simulink model "dirdyna_OffRoadRobot"  (Simulink 8.1)
settings: Solver=ode45  StartTime=0.0  StopTime=10.0  MaxStep=1e-2  RelTol=1e-3  AbsTol=1e-6
undefined symbols (not defined in the file or in its folder): Function_dirdynared, MBStoAnimFile_StopFcnCallback, Modules, Robotran, S
settings Model: Creator=habra  LastModifiedBy=habra
settings SolverCC: InitialStep=1e-3
settings DataIOCC: SignalLoggingSaveFormat=Dataset
settings OptimizationCC: ExpressionDepthLimit=128
settings DebuggingCC: FcnCallInpInsideContextMsg=EnableAllAsError
settings GRTTargetCC: CombineOutputUpdateFcns=on  GRTInterface=off

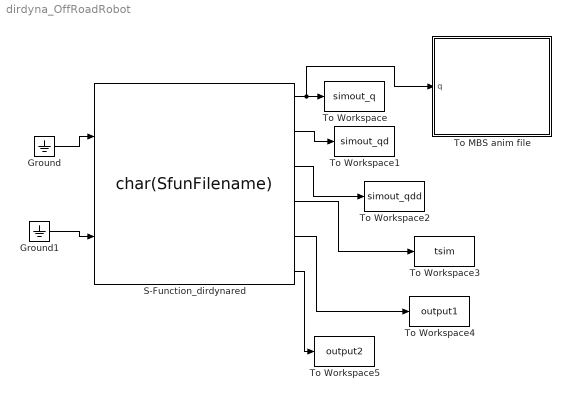
== system dirdyna_OffRoadRobot ==
  Ground : Ground
  Ground1 : Ground
  S-Function_dirdynared : S-Function  AncestorBlock=Robotran/Modules/S-Function_dirdynared  FunctionName=char(SfunFilename)  Parameters=getfield(get(gcbh,'UserData'),'mbs_data') q_ini  EnableBusSupport=off  mask(S-function: Robotran Direct Dynamics (dirdynared)){SfunFilename=mbs_sf_dirdynared_OffRoadRobot, q_ini=off, creation_date=06-May-2014}
      mask prompts: SfunFilename "S-function filename"; q_ini "Get initial qu from block inputs"; creation_date "Enter the creation date:"
      mask help: Compute the Direct Dynamics equations using symbolic MBS formalism
      settings: OpenFcn=MBSdirdynaredSfunction
      settings: CopyFcn=|
      | MBSdirdynaredSfunction;
      | set_param(gcs,'MaxStep','1e-2');
      | set_param(gcs,'InitialStep','1e-3');
      | set_param(gcs,'RelTol','1e-3');
      | set_param(gcs,'AbsTol','1e-6');
      | set_param(gcb,'OpenFcn','MBSdirdynaredSfunction');
      | set_param(gcb,'creation_date',date);
      mask Display:
      | disp('Robotran\nDirect\nDynamics\n(dirdynared)\n-\n OffRoadRobot\n-\n06-May-2014');
      | port_label('input',1,'Joint forces');
      | port_label('input',2,'Driven joints');
      | port_label('output',1,'q');
      | port_label('output',2,'qd');
      | port_label('output',3,'qdd');
  To MBS anim file : Subsystem  AncestorBlock=Robotran/Utilities/To MBS anim file  StopFcn=MBStoAnimFile_StopFcnCallback;  mask{varname=tqres, filename=simdir.anim, prjname=OffRoadRobot, overwrite=0, samplingRate=1000}
      mask prompts: varname "variable name"; filename "anim file name"; prjname "project name"; samplingRate "sampling rate"
      settings: CopyFcn=MBStoAnimFile_v2;  OpenFcn=MBStoAnimFile_v2;
      mask Display: image(imread('Logo_anim.jpg'))
  To Workspace : ToWorkspace  VariableName=simout_q  SampleTime=-1  SaveFormat=Timeseries
  To Workspace1 : ToWorkspace  VariableName=simout_qd  SampleTime=-1  SaveFormat=Timeseries
  To Workspace2 : ToWorkspace  VariableName=simout_qdd  SampleTime=-1  SaveFormat=Timeseries
  To Workspace3 : ToWorkspace  VariableName=tsim  SampleTime=-1  SaveFormat=Timeseries
  To Workspace4 : ToWorkspace  VariableName=output1  SampleTime=-1  SaveFormat=Timeseries
  To Workspace5 : ToWorkspace  VariableName=output2  SampleTime=-1  SaveFormat=Timeseries
  wires:
  Ground/1 -> S-Function_dirdynared/1
  Ground1/1 -> S-Function_dirdynared/2
  S-Function_dirdynared/1 -> To MBS anim file/1(q), To Workspace/1
  S-Function_dirdynared/2 -> To Workspace1/1
  S-Function_dirdynared/3 -> To Workspace2/1
  S-Function_dirdynared/4 -> To Workspace3/1
  S-Function_dirdynared/5 -> To Workspace4/1
  S-Function_dirdynared/6 -> To Workspace5/1

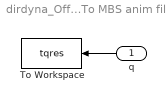
== system dirdyna_OffRoadRobot/To MBS anim file ==
  q : Inport
  To Workspace : ToWorkspace  VariableName=tqres  SampleTime=-1  SaveFormat=Structure With Time
  wires:
  q/1 -> To Workspace/1
